simulink model "RLtrot"  (R2021b)
settings: Solver=ode15s  StartTime=0.0  StopTime=Tf  FixedStep=0.01  MaxStep=0.05  RelTol=0.5  AbsTol=0.5
model workspace (MATLAB code in the model file):
  | %---------------Critical values---------------%
  | angle_amp = pi/6; % Motor rotate amplitude, ref: pi/4
  | rotateCorrectionCoef = 1.158;
  | criticalFn = 2;
  | 
  | %------values for normalization---------------%
  | % values got by running manual gait
  | rotxNormGain = 1/0.1;
  | rotyNormGain = 1/0.05;
  | rotzNormGain = 1/0.1;
  | 
  | vxNormGain = 1/0.2;
  | vyNormGain = 1/0.2;
  | vzNormGain = 1/0.2;
  | 
  | FnNormGain = 1/15;
  | 
  | %--------values for check done---------------%
  | rotDone = 0.15;
  | legBendDone = pi/3; % actuator max bending angle
  | 
  | 
  | %---------------Robot parameters-------------%
  | % robot size
  | robot_width = 0.15;
  | robot_length = 0.22;
  | 
  | % floor parameters
  | floor_length = 2;
  | floor_width = 2;
  | 
  | % continuum actuator size
  | L_disk = 0.02944;% Disk side length (m)
  | R_w = L_disk/sqrt(3);
  | thickness_disk = 0.004; % Disk thickness (m)
  | thigh_length = 0.06;
  | R_core = 0.005; % Core radius (m)
  | length_core = 0.008; % Core length (m)
  | R_spool = 0.021; % 0.01944; % radius of the spool
  | spool_height = 0.022+0.015;
  | R_pulley = 1e-3;
  | spool_k = 0;
  | spool_d = 0;
  | hole_d = 4e-3;
  | 
  | % Material property
  | rho_PLA = 1.24e3;
  | rho = 1.19e3; % 1.19e3; % Density (kg/m^3)
  | % use rigid joints
  | Pz_stiff = 135000;
  | Pz_damping = 500;
  | S_stiff = 0.0239;
  | S_damping = 7.5e-5;
  | S_low_Bound = -20;
  | S_up_Bound = 20;
  | 
  | R_foot = 0.015; % foot radius (m)
  | 
  | % motor parameter
  | stall_T = 11.2; % 11.2 cm*kg, stall torque
  | t_60_deg = 0.2; % 0.09 s
  | V_nomrmal = 6; % corresponding normal voltage
  | Jr = 0.0001; %g*cm^2, robot inertia
  | 
  | % contact force
  | coef_static_friction = 0.315;
  | coef_dynamic_friction = 0.3;
  | crictic_velocity = 0.3; % m/s
  | contact_suf_stiff = 1000; % N/m
  | contact_suf_damp = 50; % N/(m/s)
  | contact_region_width = 2e-3; % m
  | spoolOpacity = 0;
  | tendonColor = [0.902 0.902 0.902];
  | tendonOpacity = 0.1;
  | 
  | % If use point masses
  | MMainFrame = 198; % g
  | MServoMotor = 50.55;
  | MMotorSupport = 12.1;
  | MSpool = 9.2;
  | 
  | % Robot total weight about 2 kg
  | MComposateLoad = 200;
  | 
  | MBuck = 40; % x2
  | MPCB_RPi = 141.3;
  | MLiBattery = 120; % x2
  | MPowerBank = 66.5;
  | isLoadVisible = 0.1;
  | 
  | 
  | MThigh = 26.7963;
  | MCore = 0.747699;
  | MDisk = 1.78642;
  | MFoot = 16.8232;
values from neighbouring files (symbols this model uses):
  Tf = 10    [longTest.m]    (also in singleTest.m)
  Ts = 0.05    [longTest.m]    (also in singleTest.m)
  x_norm_min = min(x,[],1)    [preprocessData.m]
  x_norm_range = max(x,[],1) - min(x,[],1)    [preprocessData.m]
  y_norm_min = min(y,[],1)    [preprocessData.m]
  y_norm_range = max(y,[],1) - min(y,[],1)    [preprocessData.m]
undefined symbols (not defined in the file or in its folder): alpha_b_gain, alpha_r_gain, EntropyList, EntropyWeightList, fnVariance, isCheckDone, isContactBoolean, isUseExtAct, rotVariance, speedVariance, startAgentTime, VRef, z_l_gain
libraries: simulink x8, rllib x1, deeplib x1
settings Model: Creator=Qinglei Ji  LastModifiedBy=4DLab5
settings SolverCC: AutoScaleAbsTol=off  MaxConsecutiveZCs=100  MaxConsecutiveMinStep=10  DaesscMode=Fast  AutoInsertRateTranBlk=on
settings ExplorerConfigSet: InternalSimMechanicsExplorerSettings="<ExplorerConfiguration><canonicalview>default</canonicalview><AnimationSetting><BasePlaybackSpeed>1.0</BasePlaybackSpeed><PlaybackSpeedFactor>1.0</PlaybackSpeedFactor></AnimationSetting><TilePanel><TileInfo><Tiles Columns=\"1\" Count=\"1\" Rows=\"1\"><Column Weight=\"1\"/><Row Weight=\"1\"/><Tile Height=\"1\" Width=\"1\" X=\"0\" Y=\"0\"/></Tiles></TileInfo><SceneInfo><SceneViewer><BGColor><R>0.60000002384185791</R><G>0.60000002384185791</G><B>0.60000002384185791</B></BGColor><Camera><DoPerspective>off</DoPerspective><Position><X>-18.8331461547739707</X><Y>25.880517186070815</Y><Z>26.8100820833696147</Z></Position><Center><X>0.29785977478998571</X><Y>-0.293010908258582892</Y><Z>-0.346783787749327221</Z></Center><Up><X>0.517886432622382209</X><Y>-0.40389178028612327</Y><Z>0.754098848111419029</Z></Up><ViewLimDist>1</ViewLimDist><YLim>0.421333194645766129</YLim><XLim>0.456755011894746488</XLim></Camera></SceneViewer></SceneInfo></TilePanel><MechEditorPanel><Cameras/><GfxPanelCameraMap/><VideoCreator><PlaybackSpeedRatio>1.0</PlaybackSpeedRatio><FrameRate>60</FrameRate><VideoFormat>MPEG-4</VideoFormat><FrameSize>auto</FrameSize></VideoCreator></MechEditorPanel></ExplorerConfiguration>"

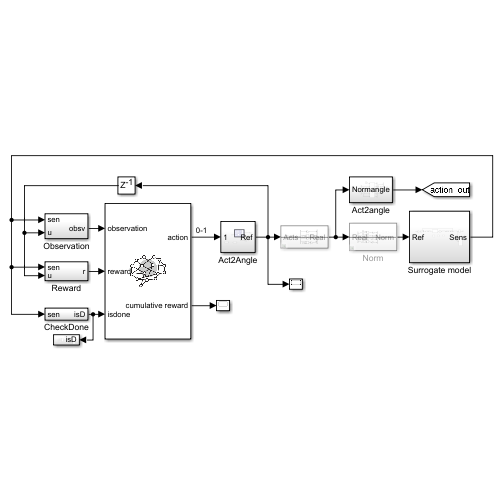
[thumbnail: Simulink's stored preview of the top-level diagram]
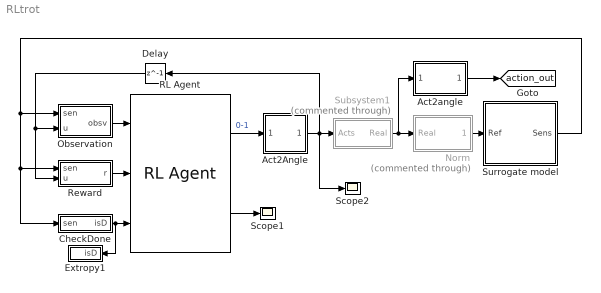
== system RLtrot ==
  Act2Angle : Subsystem
  Act2angle : Subsystem
  CheckDone : Subsystem
  Delay : Delay  DelayLength=1  InitialCondition=[0.5;0.5;0.5;0.5]
  Extropy1 : Subsystem
  Norm : Subsystem  Commented=through
  Observation : Subsystem
  RL Agent : rllib/RL Agent  Agent=agent  ExternalActionAsInput=off  ProvideCumRwd=on  TreatAsDirectFeedthrough=on
  Reward : Subsystem
  Scope1 : Scope
  Scope2 : Scope
  Subsystem1 : Subsystem  Commented=through
  Surrogate model : Subsystem
  tag scope: action_out=global
  wires:
  RL Agent/1 -> Act2Angle/1(In1)  "0-1"
  RL Agent/2 -> Scope1/1
  CheckDone/1(isD) -> Extropy1/1(isD), RL Agent/3
  Observation/1(obsv) -> RL Agent/1
  Reward/1(r) -> RL Agent/2
  Surrogate model/1(Sens) -> Observation/1(sen), Reward/1(sen), CheckDone/1(sen)
  Delay/1 -> Reward/2(u), Observation/2(u)
  Subsystem1/1(Real) -> Act2angle/1(Norm), Norm/1(Real)
  Act2Angle/1(Ref) -> Scope2/1, Delay/1, Subsystem1/1(Acts)
  Norm/1(Norm) -> Surrogate model/1(Ref)
  Act2angle/1(angle) -> [action_out]

== system RLtrot/Act2Angle ==
  note: Learn motor ref
  In1 : Inport
  DecideToUseExt : Subsystem
  Human expert : Subsystem
  Init : Subsystem
  Scope : Scope
  Subsystem2 : Subsystem  Commented=on
  action2angle : Subsystem  Commented=on
  useExt? : Switch  Criteria=u2 > Threshold
  Ref : Outport
  wires:
  In1/1 -> Init/1(In1)  "Acts"
  useExt?/1 -> Ref/1
  Human expert/1(Out1) -> useExt?/1
  DecideToUseExt/1(Out1) -> Scope/1, useExt?/2
  Init/1(Out1) -> useExt?/3

== system RLtrot/Act2angle ==
  Norm : Inport
  Demux : Demux
  MATLAB Function : MATLAB Function  TreatAsAtomicUnit=on
  MATLAB Function1 : MATLAB Function  TreatAsAtomicUnit=on
  Mux2 : Mux  Inputs=3
  Mux3 : Mux
  Mux4 : Mux  Inputs=3
  Subsystem : Subsystem
  alpha_r : Constant  Value=0
  alpha_r1 : Constant  Value=0
  angle : Outport
  wires:
  Mux2/1 -> Mux3/4, Mux3/2
  Mux4/1 -> Mux3/1, Mux3/3
  MATLAB Function1/1(alpha_A) -> Mux2/1
  MATLAB Function1/2(alpha_B) -> Mux2/2
  Mux3/1 -> angle/1  "ref"
  MATLAB Function/3(alpha_C) -> Mux4/3
  MATLAB Function/1(alpha_A) -> Mux4/1
  MATLAB Function/2(alpha_B) -> Mux4/2
  MATLAB Function1/3(alpha_C) -> Mux2/3
  alpha_r/1 -> MATLAB Function/1(alpha_r)
  alpha_r1/1 -> MATLAB Function1/1(alpha_r)
  Demux/1 -> MATLAB Function/2(alpha_b)  "b1"
  Demux/2 -> MATLAB Function/3(z_l)  "z1"
  Demux/3 -> MATLAB Function1/2(alpha_b)  "b2"
  Demux/4 -> MATLAB Function1/3(z_l)  "z2"
  Norm/1 -> Subsystem/1(Norm)
  Subsystem/1(Denorm) -> Demux/1

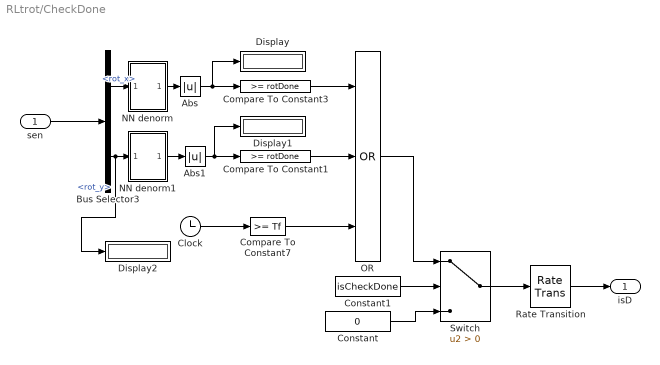
== system RLtrot/CheckDone ==
  sen : Inport
  Abs : Abs
  Abs1 : Abs
  Bus Selector3 : BusSelector  OutputSignals=rot_x,rot_y
  Clock : Clock
  Compare To Constant1 : simulink/Logic and Bit Operations/Compare To Constant  relop=>=  const=rotDone  OutDataTypeStr=boolean
  Compare To Constant3 : simulink/Logic and Bit Operations/Compare To Constant  relop=>=  const=rotDone  OutDataTypeStr=boolean
  Compare To Constant7 : simulink/Logic and Bit Operations/Compare To Constant  relop=>=  const=Tf  OutDataTypeStr=boolean
  Constant : Constant  Value=0
  Constant1 : Constant  Value=isCheckDone
  Display : Display
  Display1 : Display
  Display2 : Display
  NN denorm : Subsystem
  NN denorm1 : Subsystem
  OR : Logic  Operator=OR  Inputs=3  AllPortsSameDT=off  OutDataTypeStr=boolean
  Rate Transition : RateTransition
  Switch : Switch  Criteria=u2 > Threshold
  isD : Outport  VectorParamsAs1DForOutWhenUnconnected=off
  wires:
  sen/1 -> Bus Selector3/1
  Abs1/1 -> Display1/1, Compare To Constant1/1
  OR/1 -> Switch/1
  Compare To Constant7/1 -> OR/3
  Clock/1 -> Compare To Constant7/1
  Constant1/1 -> Switch/2
  Compare To Constant1/1 -> OR/2
  Abs/1 -> Display/1, Compare To Constant3/1
  Constant/1 -> Switch/3
  Switch/1 -> Rate Transition/1
  Compare To Constant3/1 -> OR/1
  Rate Transition/1 -> isD/1
  Bus Selector3/1 -> NN denorm/1(In1)  "<rot_x>"
  NN denorm/1(Out1) -> Abs/1
  Bus Selector3/2 -> Display2/1, NN denorm1/1(In1)  "<rot_y>"
  NN denorm1/1(Out1) -> Abs1/1

== system RLtrot/Extropy1 ==
  isD : Inport
  Clock : Clock
  Constant : Constant  Value=EntropyWeightList  SampleTime=Ts
  Constant2 : Constant  Value=EntropyList  SampleTime=Ts
  MATLAB Function : MATLAB Function  TreatAsAtomicUnit=on  SystemSampleTime=Ts
  MATLAB Function1 : MATLAB Function  TreatAsAtomicUnit=on
  wires:
  Constant2/1 -> MATLAB Function/2(EntropyList)  "entropy"
  Constant/1 -> MATLAB Function/1(EntropyWeightList)  "entroWeight"
  isD/1 -> MATLAB Function/3(isDone)
  [obsv_out] -> MATLAB Function1/2(obsv)
  [action_out] -> MATLAB Function1/3(act)
  Clock/1 -> MATLAB Function1/1(time)

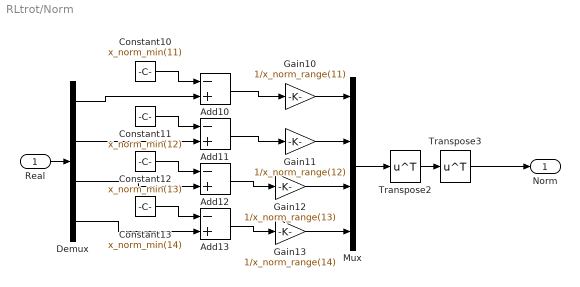
== system RLtrot/Norm ==
  Real : Inport
  Add{10..13} (4 alike) : Sum  Inputs=-+
  Constant10 : Constant  Value=x_norm_min(11)
  Constant11 : Constant  Value=x_norm_min(12)
  Constant12 : Constant  Value=x_norm_min(13)
  Constant13 : Constant  Value=x_norm_min(14)
  Demux : Demux
  Gain10 : Gain  Gain=1/x_norm_range(11)
  Gain11 : Gain  Gain=1/x_norm_range(12)
  Gain12 : Gain  Gain=1/x_norm_range(13)
  Gain13 : Gain  Gain=1/x_norm_range(14)
  Mux : Mux
  Transpose2 : Math  Operator=transpose  SaturateOnIntegerOverflow=on
  Transpose3 : Math  Operator=transpose  SaturateOnIntegerOverflow=on
  Norm : Outport
  wires:
  Constant10/1 -> Add10/1
  Constant11/1 -> Add11/1
  Demux/2 -> Add11/2
  Gain13/1 -> Mux/4
  Demux/4 -> Add13/2
  Add12/1 -> Gain12/1
  Demux/1 -> Add10/2
  Gain11/1 -> Mux/2
  Gain12/1 -> Mux/3
  Add11/1 -> Gain11/1
  Constant12/1 -> Add12/1
  Add10/1 -> Gain10/1
  Constant13/1 -> Add13/1
  Demux/3 -> Add12/2
  Add13/1 -> Gain13/1
  Gain10/1 -> Mux/1
  Real/1 -> Demux/1
  Transpose2/1 -> Transpose3/1
  Transpose3/1 -> Norm/1
  Mux/1 -> Transpose2/1

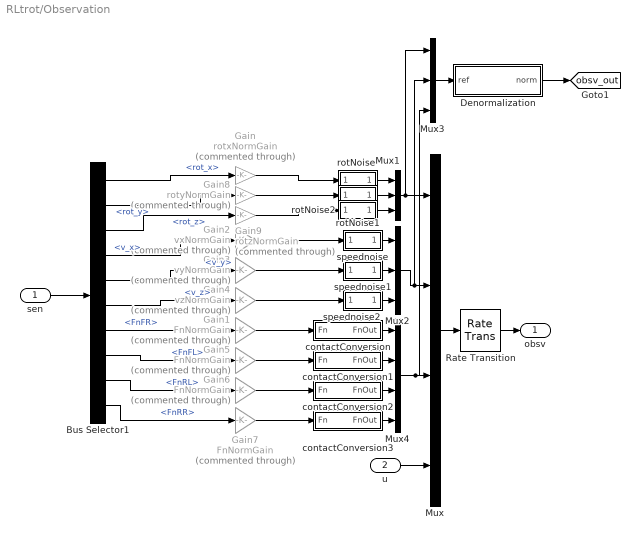
== system RLtrot/Observation ==
  sen : Inport
  u : Inport  Port=2
  Bus Selector1 : BusSelector  OutputSignals=rot_x,rot_y,rot_z,v_x,v_y,v_z,FnFR,FnFL,FnRL,FnRR
  Denormalization : Subsystem
  Gain : Gain  Commented=through  Gain=rotxNormGain
  Gain{1,5..7} (4 alike) : Gain  Commented=through  Gain=FnNormGain
  Gain2 : Gain  Commented=through  Gain=vxNormGain
  Gain3 : Gain  Commented=through  Gain=vyNormGain
  Gain4 : Gain  Commented=through  Gain=vzNormGain
  Gain8 : Gain  Commented=through  Gain=rotyNormGain
  Gain9 : Gain  Commented=through  Gain=rotzNormGain
  Mux : Mux
  Mux1 : Mux  Inputs=3
  Mux2 : Mux  Inputs=3
  Mux3 : Mux  Inputs=3
  Mux4 : Mux
  Rate Transition : RateTransition  OutPortSampleTime=Ts
  contactConversion : Subsystem
  contactConversion1 : Subsystem
  contactConversion2 : Subsystem
  contactConversion3 : Subsystem
  rotNoise : Subsystem
  rotNoise1 : Subsystem
  rotNoise2 : Subsystem
  speednoise : Subsystem
  speednoise1 : Subsystem
  speednoise2 : Subsystem
  obsv : Outport  VectorParamsAs1DForOutWhenUnconnected=off
  tag scope: obsv_out=global
  wires:
  Mux/1 -> Rate Transition/1
  sen/1 -> Bus Selector1/1
  Rate Transition/1 -> obsv/1
  u/1 -> Mux/4
  Mux1/1 -> Mux3/1, Mux/1
  Mux2/1 -> Mux3/2, Mux/2
  contactConversion/1(FnOut) -> Mux4/1
  contactConversion1/1(FnOut) -> Mux4/2
  contactConversion2/1(FnOut) -> Mux4/3
  contactConversion3/1(FnOut) -> Mux4/4
  Mux4/1 -> Mux3/3, Mux/3
  speednoise/1(Out1) -> Mux2/1
  speednoise1/1(Out1) -> Mux2/2
  speednoise2/1(Out1) -> Mux2/3
  Bus Selector1/1 -> Gain/1  "<rot_x>"
  rotNoise/1(Out1) -> Mux1/1
  rotNoise1/1(Out1) -> Mux1/2
  rotNoise2/1(Out1) -> Mux1/3
  Bus Selector1/2 -> Gain8/1  "<rot_y>"
  Bus Selector1/3 -> Gain9/1  "<rot_z>"
  Bus Selector1/4 -> Gain2/1  "<v_x>"
  Bus Selector1/5 -> Gain3/1  "<v_y>"
  Bus Selector1/6 -> Gain4/1  "<v_z>"
  Bus Selector1/7 -> Gain1/1  "<FnFR>"
  Bus Selector1/8 -> Gain5/1  "<FnFL>"
  Bus Selector1/9 -> Gain6/1  "<FnRL>"
  Bus Selector1/10 -> Gain7/1  "<FnRR>"
  Gain/1 -> rotNoise/1(<vx>)
  Gain8/1 -> rotNoise1/1(<vx>)
  Gain9/1 -> rotNoise2/1(<vx>)
  Gain2/1 -> speednoise/1(<vx>)
  Gain1/1 -> contactConversion/1(Fn)
  Gain6/1 -> contactConversion2/1(Fn)
  Gain5/1 -> contactConversion1/1(Fn)
  Gain3/1 -> speednoise1/1(<vx>)
  Gain4/1 -> speednoise2/1(<vx>)
  Gain7/1 -> contactConversion3/1(Fn)
  Denormalization/1(norm) -> [obsv_out]
  Mux3/1 -> Denormalization/1(ref)

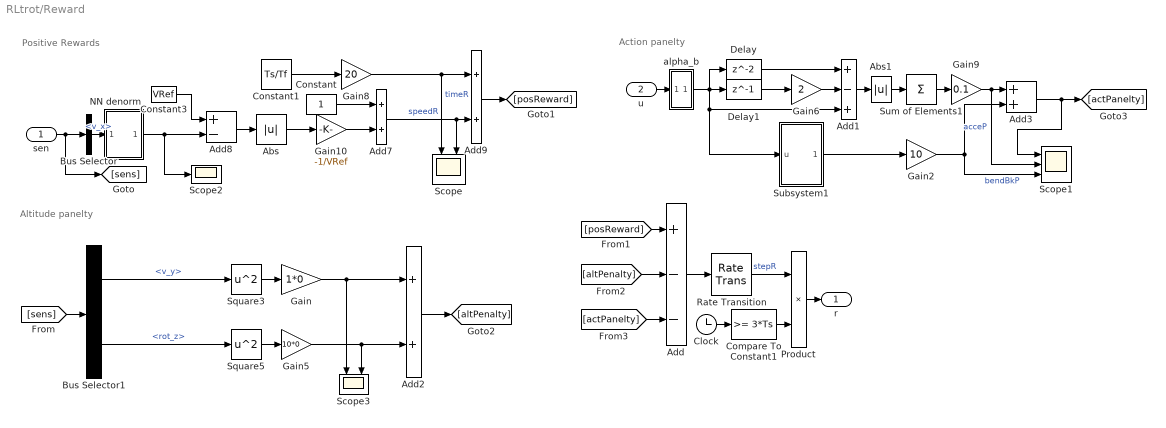
== system RLtrot/Reward ==
  note: Action panelty
  note: Altitude panelty
  note: Positive Rewards
  sen : Inport
  u : Inport  Port=2
  Abs : Abs
  Abs1 : Abs
  Add : Sum  Inputs=+--
  Add1 : Sum  Inputs=+-+
  Add{2..3,7,9} (4 alike) : Sum
  Add8 : Sum  Inputs=+-
  Bus Selector : BusSelector  OutputSignals=v_x
  Bus Selector1 : BusSelector  OutputSignals=v_y,rot_z
  Clock : Clock
  Compare To Constant1 : simulink/Logic and Bit Operations/Compare To Constant  relop=>=  const=3*Ts  OutDataTypeStr=boolean
  Constant : Constant
  Constant1 : Constant  Value=Ts/Tf
  Constant3 : Constant  Value=VRef
  Delay : Delay  InitialCondition=0.5
  Delay1 : Delay  DelayLength=1  InitialCondition=0.5
  Gain : Gain  Gain=1*0
  Gain10 : Gain  Gain=-1/VRef
  Gain2 : Gain  Gain=10
  Gain5 : Gain  Gain=10*0
  Gain6 : Gain  Gain=2
  Gain8 : Gain  Gain=20
  Gain9 : Gain  Gain=0.1
  NN denorm : Subsystem
  Product : Product
  Rate Transition : RateTransition  OutPortSampleTime=Ts
  Scope : Scope  NumInputPorts=2
  Scope1 : Scope  NumInputPorts=3
  Scope2 : Scope
  Scope3 : Scope  NumInputPorts=2
  Square3 : Math  Operator=square  SignedPower=on  SaturateOnIntegerOverflow=on
  Square5 : Math  Operator=square  SignedPower=on  SaturateOnIntegerOverflow=on
  Subsystem1 : Subsystem
  Sum of Elements1 : Sum  Inputs=+
  alpha_b : Subsystem
  r : Outport  VectorParamsAs1DForOutWhenUnconnected=off
  wires:
  sen/1 -> Bus Selector/1, [sens]
  Square3/1 -> Gain/1
  Square5/1 -> Gain5/1
  Bus Selector1/2 -> Square5/1  "<rot_z>"
  Gain/1 -> Scope3/1, Add2/1
  Add/1 -> Rate Transition/1
  Constant1/1 -> Gain8/1
  Delay/1 -> Add1/1
  Gain6/1 -> Add1/2
  Add1/1 -> Abs1/1
  Abs1/1 -> Sum of Elements1/1
  Delay1/1 -> Gain6/1
  Sum of Elements1/1 -> Gain9/1
  Clock/1 -> Compare To Constant1/1
  Compare To Constant1/1 -> Product/2
  Rate Transition/1 -> Product/1  "stepR"
  Product/1 -> r/1
  [sens] -> Bus Selector1/1
  Gain8/1 -> Add9/1, Scope/1  "timeR"
  Add9/1 -> [posReward]
  Bus Selector1/1 -> Square3/1  "<v_y>"
  Gain5/1 -> Add2/2, Scope3/2
  Add2/1 -> [altPenalty]
  [posReward] -> Add/1
  [altPenalty] -> Add/2
  [actPanelty] -> Add/3
  Add8/1 -> Abs/1
  Add7/1 -> Scope/2, Add9/2  "speedR"
  Gain10/1 -> Add7/2
  Abs/1 -> Gain10/1
  Constant/1 -> Add7/1
  Constant3/1 -> Add8/1
  Bus Selector/1 -> NN denorm/1(In1)  "<v_x>"
  NN denorm/1(Out1) -> Scope2/1, Add8/2
  Gain9/1 -> Scope1/2, Add3/1  "acceP"
  Add3/1 -> Scope1/1, [actPanelty]
  u/1 -> alpha_b/1(u)
  Subsystem1/1(Out1) -> Gain2/1
  Gain2/1 -> Add3/2, Scope1/3  "bendBkP"
  alpha_b/1(b) -> Add1/3, Subsystem1/1(u), Delay/1, Delay1/1

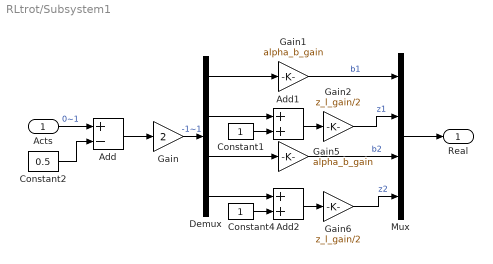
== system RLtrot/Subsystem1 ==
  Acts : Inport
  Add : Sum  Inputs=+-
  Add1 : Sum
  Add2 : Sum
  Constant1 : Constant
  Constant2 : Constant  Value=0.5
  Constant4 : Constant
  Demux : Demux
  Gain : Gain  Gain=2
  Gain1 : Gain  Gain=alpha_b_gain
  Gain2 : Gain  Gain=z_l_gain/2
  Gain5 : Gain  Gain=alpha_b_gain
  Gain6 : Gain  Gain=z_l_gain/2
  Mux : Mux
  Real : Outport
  wires:
  Demux/4 -> Add2/1
  Constant1/1 -> Add1/2
  Add1/1 -> Gain2/1
  Constant4/1 -> Add2/2
  Gain1/1 -> Mux/1  "b1"
  Acts/1 -> Add/1  "0~1"
  Constant2/1 -> Add/2
  Gain/1 -> Demux/1  "-1~1"
  Add2/1 -> Gain6/1
  Add/1 -> Gain/1
  Demux/1 -> Gain1/1
  Gain6/1 -> Mux/4  "z2"
  Mux/1 -> Real/1
  Gain2/1 -> Mux/2  "z1"
  Demux/2 -> Add1/1
  Demux/3 -> Gain5/1
  Gain5/1 -> Mux/3  "b2"

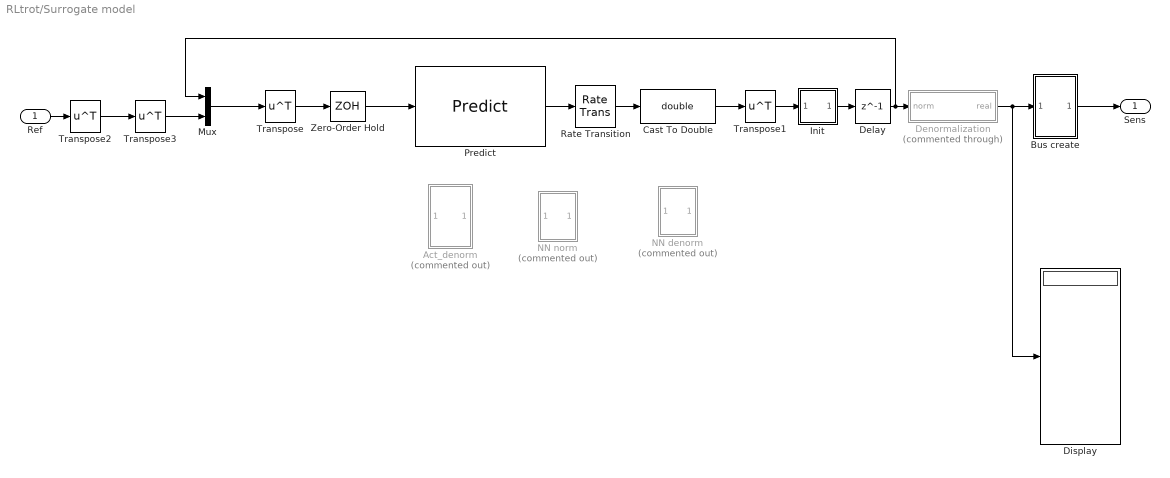
== system RLtrot/Surrogate model ==
  Ref : Inport
  Act_denorm : Subsystem  Commented=on
  Bus create : Subsystem
  Cast To Double : DataTypeConversion  OutDataTypeStr=double
  Delay : Delay  DelayLength=1  InitialCondition=x_norm_init'  SampleTime=Ts
  Denormalization : Subsystem  Commented=through
  Display : Display
  Init : Subsystem
  Mux : Mux  Inputs=2
  NN denorm : Subsystem  Commented=on
  NN norm : Subsystem  Commented=on
  Predict : deeplib/Predict  Network=Network from MAT-file  NetworkFunction=squeezenet  NetworkFilePath=C:\Users\4DLab5\OneDrive - KTH\KTH\Master Thesis\Github\MBRL23KTH\net_best.mat  MiniBatchSize=512  InputDataFormats={ 'observation', '[1x22]' }  Predictions=on  Activations={}  ForceInterpretedSim=off  EnableDLNetwork=on
      settings: SourceProductBaseCode=NN
  Rate Transition : RateTransition  OutPortSampleTime=Ts
  Transpose{,1..3} (4 alike) : Math  Operator=transpose  SaturateOnIntegerOverflow=on
  Zero-Order Hold : ZeroOrderHold  SampleTime=Ts
  Sens : Outport  OutDataTypeStr=double
  wires:
  Predict/1 -> Rate Transition/1
  Cast To Double/1 -> Transpose1/1
  Bus create/1(Outport) -> Sens/1
  Transpose/1 -> Zero-Order Hold/1
  Denormalization/1(real) -> Display/1, Bus create/1(In1)
  Mux/1 -> Transpose/1
  Init/1(Out1) -> Delay/1
  Transpose1/1 -> Init/1(In1)
  Delay/1 -> Mux/1, Denormalization/1(norm)
  Rate Transition/1 -> Cast To Double/1
  Zero-Order Hold/1 -> Predict/1
  Transpose2/1 -> Transpose3/1
  Transpose3/1 -> Mux/2
  Ref/1 -> Transpose2/1

== system RLtrot/Act2Angle/DecideToUseExt ==
  Clock : Clock
  Constant : Constant  Value=isUseExtAct
  Constant1 : Constant  Value=0
  Constant2 : Constant
  Constant3 : Constant  Value=0
  Switch : Switch  Criteria=u2 > Threshold  Threshold=startAgentTime
  Switch1 : Switch  Criteria=u2 > Threshold
  Out1 : Outport
  wires:
  Constant/1 -> Switch1/2
  Switch1/1 -> Out1/1
  Constant2/1 -> Switch/3
  Constant1/1 -> Switch/1
  Clock/1 -> Switch/2
  Constant3/1 -> Switch1/3
  Switch/1 -> Switch1/1

== system RLtrot/Act2Angle/Human expert ==
  Mux10 : Mux
  alpha_b : simulink/Sources/Repeating Sequence  rep_seq_t=[0 0.2 0.4 0.6 0.8]  rep_seq_y=[0.5 1 0.5 0 0.5]
  alpha_b1 : simulink/Sources/Repeating Sequence  rep_seq_t=[0 0.2 0.4 0.6 0.8]  rep_seq_y=[0.5 0 0.5 1 0.5]
  z_l : simulink/Sources/Repeating Sequence  rep_seq_t=[0 0.2 0.4 0.6 0.8]  rep_seq_y=[0 1 1 1 0]
  z_l1 : simulink/Sources/Repeating Sequence  rep_seq_t=[0 0.2 0.4 0.6 0.8]  rep_seq_y=[1 1 0 1 1]
  Out1 : Outport
  wires:
  Mux10/1 -> Out1/1
  alpha_b/1 -> Mux10/1  "alpha_b_Ref"
  z_l1/1 -> Mux10/4  "z_l_Ref"
  z_l/1 -> Mux10/2  "z_l_Ref"
  alpha_b1/1 -> Mux10/3  "alpha_b_Ref"

== system RLtrot/Act2Angle/Init ==
  In1 : Inport
  Clock : Clock
  Constant{6..9} (4 alike) : Constant  Value=0.5
  Initial : Switch  Threshold=Ts
  Mux : Mux
  Out1 : Outport
  wires:
  Mux/1 -> Initial/3
  In1/1 -> Initial/1
  Initial/1 -> Out1/1  "prosedAct"
  Clock/1 -> Initial/2
  Constant9/1 -> Mux/4
  Constant6/1 -> Mux/1
  Constant8/1 -> Mux/3
  Constant7/1 -> Mux/2

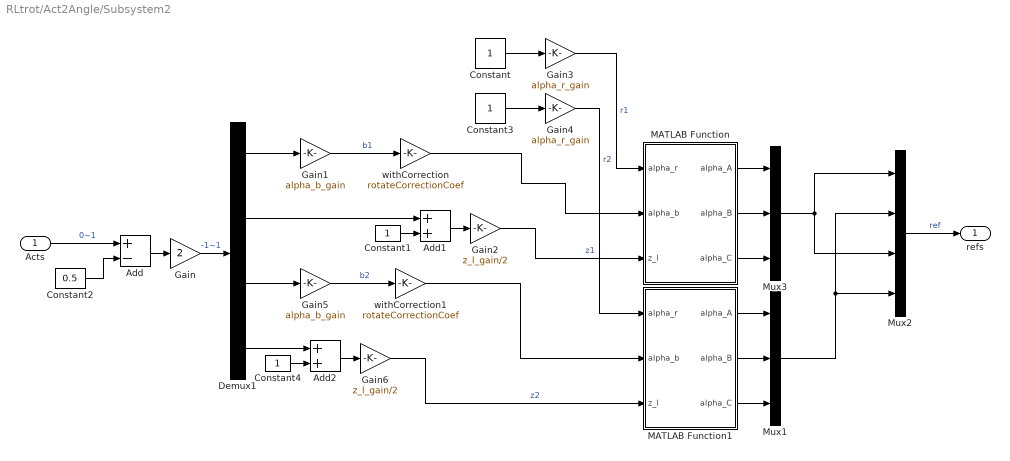
== system RLtrot/Act2Angle/Subsystem2 ==
  Acts : Inport
  Add : Sum  Inputs=+-
  Add1 : Sum
  Add2 : Sum
  Constant{,1,3..4} (4 alike) : Constant
  Constant2 : Constant  Value=0.5
  Demux1 : Demux
  Gain : Gain  Gain=2
  Gain1 : Gain  Gain=alpha_b_gain
  Gain2 : Gain  Gain=z_l_gain/2
  Gain3 : Gain  Gain=alpha_r_gain
  Gain4 : Gain  Gain=alpha_r_gain
  Gain5 : Gain  Gain=alpha_b_gain
  Gain6 : Gain  Gain=z_l_gain/2
  MATLAB Function : MATLAB Function  TreatAsAtomicUnit=on
  MATLAB Function1 : MATLAB Function  TreatAsAtomicUnit=on
  Mux1 : Mux  Inputs=3
  Mux2 : Mux
  Mux3 : Mux  Inputs=3
  withCorrection : Gain  Gain=rotateCorrectionCoef
  withCorrection1 : Gain  Gain=rotateCorrectionCoef
  refs : Outport
  wires:
  Gain6/1 -> MATLAB Function1/3(z_l)  "z2"
  Mux2/1 -> refs/1  "ref"
  Gain2/1 -> MATLAB Function/3(z_l)  "z1"
  Gain4/1 -> MATLAB Function1/1(alpha_r)  "r2"
  MATLAB Function1/1(alpha_A) -> Mux1/1
  Gain3/1 -> MATLAB Function/1(alpha_r)  "r1"
  Gain1/1 -> withCorrection/1  "b1"
  MATLAB Function/3(alpha_C) -> Mux3/3
  MATLAB Function1/3(alpha_C) -> Mux1/3
  MATLAB Function/1(alpha_A) -> Mux3/1
  MATLAB Function/2(alpha_B) -> Mux3/2
  MATLAB Function1/2(alpha_B) -> Mux1/2
  Mux3/1 -> Mux2/1, Mux2/3
  Mux1/1 -> Mux2/4, Mux2/2
  Demux1/1 -> Gain1/1
  Constant/1 -> Gain3/1
  Constant3/1 -> Gain4/1
  Constant1/1 -> Add1/2
  Add1/1 -> Gain2/1
  Gain5/1 -> withCorrection1/1  "b2"
  Demux1/4 -> Add2/1
  Add2/1 -> Gain6/1
  Constant4/1 -> Add2/2
  withCorrection/1 -> MATLAB Function/2(alpha_b)
  withCorrection1/1 -> MATLAB Function1/2(alpha_b)
  Constant2/1 -> Add/2
  Acts/1 -> Add/1  "0~1"
  Add/1 -> Gain/1
  Gain/1 -> Demux1/1  "-1~1"
  Demux1/2 -> Add1/1
  Demux1/3 -> Gain5/1

== system RLtrot/Act2Angle/action2angle ==
  In1 : Inport
  Add : Sum  Inputs=+-
  Constant2 : Constant  Value=0.5
  withCorrection : Gain  Gain=angle_amp/0.5*rotateCorrectionCoef
  currAct_vec : Outport
  wires:
  In1/1 -> Add/1
  Constant2/1 -> Add/2
  Add/1 -> withCorrection/1
  withCorrection/1 -> currAct_vec/1

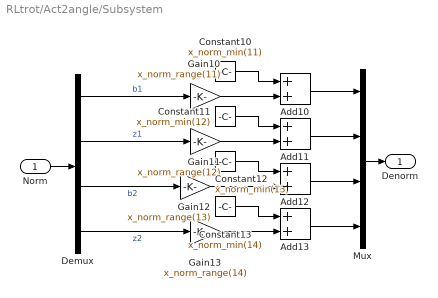
== system RLtrot/Act2angle/Subsystem ==
  Norm : Inport
  Add{10..13} (4 alike) : Sum
  Constant10 : Constant  Value=x_norm_min(11)
  Constant11 : Constant  Value=x_norm_min(12)
  Constant12 : Constant  Value=x_norm_min(13)
  Constant13 : Constant  Value=x_norm_min(14)
  Demux : Demux
  Gain10 : Gain  Gain=x_norm_range(11)
  Gain11 : Gain  Gain=x_norm_range(12)
  Gain12 : Gain  Gain=x_norm_range(13)
  Gain13 : Gain  Gain=x_norm_range(14)
  Mux : Mux
  Denorm : Outport
  wires:
  Constant12/1 -> Add12/1
  Add13/1 -> Mux/4
  Gain10/1 -> Add10/2
  Gain11/1 -> Add11/2
  Demux/1 -> Gain10/1  "b1"
  Add11/1 -> Mux/2
  Demux/3 -> Gain12/1  "b2"
  Gain13/1 -> Add13/2
  Gain12/1 -> Add12/2
  Constant13/1 -> Add13/1
  Mux/1 -> Denorm/1
  Demux/4 -> Gain13/1  "z2"
  Add10/1 -> Mux/1
  Add12/1 -> Mux/3
  Constant11/1 -> Add11/1
  Demux/2 -> Gain11/1  "z1"
  Constant10/1 -> Add10/1
  Norm/1 -> Demux/1

== system RLtrot/CheckDone/NN denorm ==
  In1 : Inport
  0~1to-1~1s : Subsystem  Commented=through
  Add : Sum
  Constant : Constant  Value=y_norm_min(1)  SampleTime=Ts
  Gain : Gain  Gain=y_norm_range(1)
  Out1 : Outport
  wires:
  Constant/1 -> Add/2
  Add/1 -> Out1/1
  Gain/1 -> Add/1
  In1/1 -> 0~1to-1~1s/1(In1)
  0~1to-1~1s/1(Out1) -> Gain/1

== system RLtrot/CheckDone/NN denorm1 ==
  In1 : Inport
  0~1to-1~1s : Subsystem  Commented=through
  Add : Sum
  Constant : Constant  Value=y_norm_min(2)  SampleTime=Ts
  Gain : Gain  Gain=y_norm_range(2)
  Out1 : Outport
  wires:
  Constant/1 -> Add/2
  Add/1 -> Out1/1
  Gain/1 -> Add/1
  In1/1 -> 0~1to-1~1s/1(In1)
  0~1to-1~1s/1(Out1) -> Gain/1

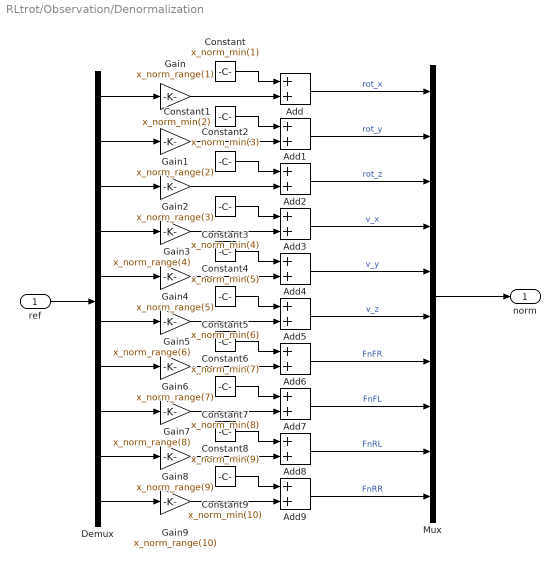
== system RLtrot/Observation/Denormalization ==
  ref : Inport
  Add{,1..9} (10 alike) : Sum
  Constant : Constant  Value=x_norm_min(1)
  Constant1 : Constant  Value=x_norm_min(2)
  Constant2 : Constant  Value=x_norm_min(3)
  Constant3 : Constant  Value=x_norm_min(4)
  Constant4 : Constant  Value=x_norm_min(5)
  Constant5 : Constant  Value=x_norm_min(6)
  Constant6 : Constant  Value=x_norm_min(7)
  Constant7 : Constant  Value=x_norm_min(8)
  Constant8 : Constant  Value=x_norm_min(9)
  Constant9 : Constant  Value=x_norm_min(10)
  Demux : Demux  Outputs=10
  Gain : Gain  Gain=x_norm_range(1)
  Gain1 : Gain  Gain=x_norm_range(2)
  Gain2 : Gain  Gain=x_norm_range(3)
  Gain3 : Gain  Gain=x_norm_range(4)
  Gain4 : Gain  Gain=x_norm_range(5)
  Gain5 : Gain  Gain=x_norm_range(6)
  Gain6 : Gain  Gain=x_norm_range(7)
  Gain7 : Gain  Gain=x_norm_range(8)
  Gain8 : Gain  Gain=x_norm_range(9)
  Gain9 : Gain  Gain=x_norm_range(10)
  Mux : Mux  Inputs=10
  norm : Outport
  wires:
  Mux/1 -> norm/1
  ref/1 -> Demux/1
  Constant/1 -> Add/1
  Constant1/1 -> Add1/1
  Constant2/1 -> Add2/1
  Constant3/1 -> Add3/1
  Constant4/1 -> Add4/1
  Constant5/1 -> Add5/1
  Constant6/1 -> Add6/1
  Constant7/1 -> Add7/1
  Constant8/1 -> Add8/1
  Constant9/1 -> Add9/1
  Demux/1 -> Gain/1
  Demux/2 -> Gain1/1
  Demux/3 -> Gain2/1
  Demux/4 -> Gain3/1
  Demux/5 -> Gain4/1
  Demux/6 -> Gain5/1
  Demux/7 -> Gain6/1
  Demux/8 -> Gain7/1
  Demux/9 -> Gain8/1
  Demux/10 -> Gain9/1
  Gain9/1 -> Add9/2
  Gain/1 -> Add/2
  Gain1/1 -> Add1/2
  Gain2/1 -> Add2/2
  Gain3/1 -> Add3/2
  Gain4/1 -> Add4/2
  Gain5/1 -> Add5/2
  Gain6/1 -> Add6/2
  Gain7/1 -> Add7/2
  Gain8/1 -> Add8/2
  Add/1 -> Mux/1  "rot_x"
  Add1/1 -> Mux/2  "rot_y"
  Add2/1 -> Mux/3  "rot_z"
  Add3/1 -> Mux/4  "v_x"
  Add9/1 -> Mux/10  "FnRR"
  Add8/1 -> Mux/9  "FnRL"
  Add7/1 -> Mux/8  "FnFL"
  Add6/1 -> Mux/7  "FnFR"
  Add5/1 -> Mux/6  "v_z"
  Add4/1 -> Mux/5  "v_y"

== system RLtrot/Observation/contactConversion ==
  Fn : Inport
  Constant : Constant  Value=isContactBoolean
  Constant1 : Constant
  Constant2 : Constant  Value=0
  Switch : Switch  Criteria=u2 > Threshold  Threshold=criticalFn*FnNormGain
  Switch1 : Switch  Criteria=u2 > Threshold
  fnNoise : Subsystem
  FnOut : Outport
  wires:
  Fn/1 -> fnNoise/1(<vx>)
  Constant/1 -> Switch1/2
  Constant2/1 -> Switch/3
  Constant1/1 -> Switch/1
  Switch/1 -> Switch1/1
  Switch1/1 -> FnOut/1
  fnNoise/1(Out1) -> Switch/2, Switch1/3

== system RLtrot/Observation/contactConversion1 ==
  Fn : Inport
  Constant : Constant  Value=isContactBoolean
  Constant1 : Constant
  Constant2 : Constant  Value=0
  Switch : Switch  Criteria=u2 > Threshold  Threshold=criticalFn*FnNormGain
  Switch1 : Switch  Criteria=u2 > Threshold
  fnNoise : Subsystem
  FnOut : Outport
  wires:
  Fn/1 -> fnNoise/1(<vx>)
  Constant/1 -> Switch1/2
  Constant2/1 -> Switch/3
  Constant1/1 -> Switch/1
  Switch/1 -> Switch1/1
  Switch1/1 -> FnOut/1
  fnNoise/1(Out1) -> Switch/2, Switch1/3

== system RLtrot/Observation/contactConversion2 ==
  Fn : Inport
  Constant : Constant  Value=isContactBoolean
  Constant1 : Constant
  Constant2 : Constant  Value=0
  Switch : Switch  Criteria=u2 > Threshold  Threshold=criticalFn*FnNormGain
  Switch1 : Switch  Criteria=u2 > Threshold
  fnNoise : Subsystem
  FnOut : Outport
  wires:
  Fn/1 -> fnNoise/1(<vx>)
  Constant/1 -> Switch1/2
  Constant2/1 -> Switch/3
  Constant1/1 -> Switch/1
  Switch/1 -> Switch1/1
  Switch1/1 -> FnOut/1
  fnNoise/1(Out1) -> Switch/2, Switch1/3

== system RLtrot/Observation/contactConversion3 ==
  Fn : Inport
  Constant : Constant  Value=isContactBoolean
  Constant1 : Constant
  Constant2 : Constant  Value=0
  Switch : Switch  Criteria=u2 > Threshold  Threshold=criticalFn*FnNormGain
  Switch1 : Switch  Criteria=u2 > Threshold
  fnNoise : Subsystem
  FnOut : Outport
  wires:
  Fn/1 -> fnNoise/1(<vx>)
  Constant/1 -> Switch1/2
  Constant2/1 -> Switch/3
  Constant1/1 -> Switch/1
  Switch/1 -> Switch1/1
  Switch1/1 -> FnOut/1
  fnNoise/1(Out1) -> Switch/2, Switch1/3

== system RLtrot/Observation/rotNoise ==
  <vx> : Inport
  Add : Sum
  Random Number : RandomNumber  Variance=rotVariance  SampleTime=Ts
  Out1 : Outport
  wires:
  Random Number/1 -> Add/1
  <vx>/1 -> Add/2
  Add/1 -> Out1/1

== system RLtrot/Observation/rotNoise1 ==
  <vx> : Inport
  Add : Sum
  Random Number : RandomNumber  Variance=rotVariance  Seed=1  SampleTime=Ts
  Out1 : Outport
  wires:
  Random Number/1 -> Add/1
  <vx>/1 -> Add/2
  Add/1 -> Out1/1

== system RLtrot/Observation/rotNoise2 ==
  <vx> : Inport
  Add : Sum
  Random Number : RandomNumber  Variance=rotVariance  Seed=12  SampleTime=Ts
  Out1 : Outport
  wires:
  Random Number/1 -> Add/1
  <vx>/1 -> Add/2
  Add/1 -> Out1/1

== system RLtrot/Observation/speednoise ==
  <vx> : Inport
  Add : Sum
  Random Number : RandomNumber  Variance=speedVariance  Seed=3  SampleTime=Ts
  Out1 : Outport
  wires:
  Random Number/1 -> Add/1
  <vx>/1 -> Add/2
  Add/1 -> Out1/1

== system RLtrot/Observation/speednoise1 ==
  <vx> : Inport
  Add : Sum
  Random Number : RandomNumber  Variance=speedVariance  Seed=4  SampleTime=Ts
  Out1 : Outport
  wires:
  Random Number/1 -> Add/1
  <vx>/1 -> Add/2
  Add/1 -> Out1/1

== system RLtrot/Observation/speednoise2 ==
  <vx> : Inport
  Add : Sum
  Random Number : RandomNumber  Variance=speedVariance  Seed=5  SampleTime=Ts
  Out1 : Outport
  wires:
  Random Number/1 -> Add/1
  <vx>/1 -> Add/2
  Add/1 -> Out1/1

== system RLtrot/Reward/NN denorm ==
  In1 : Inport
  Add : Sum
  Constant : Constant  Value=y_norm_min(4)  SampleTime=Ts
  Gain : Gain  Gain=y_norm_range(4)
  Out1 : Outport
  wires:
  Constant/1 -> Add/2
  Add/1 -> Out1/1
  Gain/1 -> Add/1
  In1/1 -> Gain/1

== system RLtrot/Reward/Subsystem1 ==
  u : Inport
  Abs1 : Abs
  Add : Sum
  Add1 : Sum  Inputs=+-
  Add2 : Sum  Inputs=+-
  Constant : Constant  Value=2*0.35
  Constant1 : Constant  Value=4*0.36
  Constant2 : Constant  Value=0
  Demux : Demux  Outputs=2
  Math Function : Math  Operator=square  SaturateOnIntegerOverflow=on
  Max : MinMax  Function=max  Inputs=2
  Out1 : Outport
  wires:
  Math Function/1 -> Out1/1
  u/1 -> Demux/1
  Demux/1 -> Add/1  "b1"
  Demux/2 -> Add/2  "b2"
  Add/1 -> Add1/1
  Constant/1 -> Add1/2
  Add1/1 -> Abs1/1
  Abs1/1 -> Add2/1
  Constant1/1 -> Add2/2
  Add2/1 -> Max/1
  Constant2/1 -> Max/2
  Max/1 -> Math Function/1

== system RLtrot/Reward/alpha_b ==
  u : Inport
  Demux : Demux
  Mux : Mux  Inputs=2
  Terminator : Terminator
  Terminator1 : Terminator
  b : Outport
  wires:
  Demux/3 -> Mux/2  "b2"
  Demux/1 -> Mux/1  "b1"
  Demux/2 -> Terminator/1  "z1"
  Mux/1 -> b/1
  u/1 -> Demux/1
  Demux/4 -> Terminator1/1  "z2"

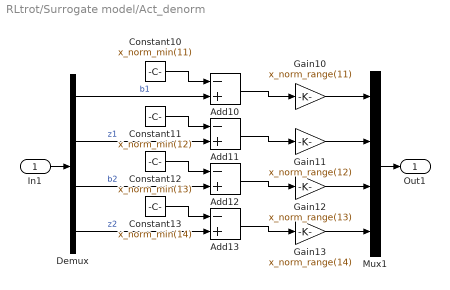
== system RLtrot/Surrogate model/Act_denorm ==
  In1 : Inport
  Add{10..13} (4 alike) : Sum  Inputs=-+
  Constant10 : Constant  Value=x_norm_min(11)
  Constant11 : Constant  Value=x_norm_min(12)
  Constant12 : Constant  Value=x_norm_min(13)
  Constant13 : Constant  Value=x_norm_min(14)
  Demux : Demux
  Gain10 : Gain  Gain=x_norm_range(11)
  Gain11 : Gain  Gain=x_norm_range(12)
  Gain12 : Gain  Gain=x_norm_range(13)
  Gain13 : Gain  Gain=x_norm_range(14)
  Mux1 : Mux
  Out1 : Outport
  wires:
  Gain11/1 -> Mux1/2
  Gain13/1 -> Mux1/4
  Gain10/1 -> Mux1/1
  Gain12/1 -> Mux1/3
  Demux/3 -> Add12/2  "b2"
  Mux1/1 -> Out1/1
  Demux/2 -> Add11/2  "z1"
  In1/1 -> Demux/1
  Demux/4 -> Add13/2  "z2"
  Demux/1 -> Add10/2  "b1"
  Add12/1 -> Gain12/1
  Constant13/1 -> Add13/1
  Add13/1 -> Gain13/1
  Add10/1 -> Gain10/1
  Constant11/1 -> Add11/1
  Constant12/1 -> Add12/1
  Add11/1 -> Gain11/1
  Constant10/1 -> Add10/1

== system RLtrot/Surrogate model/Bus create ==
  In1 : Inport
  Bus Creator : BusCreator  Inputs=10
  Demux : Demux  Outputs=10
  Outport : Outport
  wires:
  In1/1 -> Demux/1
  Demux/1 -> Bus Creator/1  "rot_x"
  Demux/2 -> Bus Creator/2  "rot_y"
  Demux/3 -> Bus Creator/3  "rot_z"
  Bus Creator/1 -> Outport/1
  Demux/4 -> Bus Creator/4  "v_x"
  Demux/5 -> Bus Creator/5  "v_y"
  Demux/6 -> Bus Creator/6  "v_z"
  Demux/7 -> Bus Creator/7  "FnFR"
  Demux/8 -> Bus Creator/8  "FnFL"
  Demux/9 -> Bus Creator/9  "FnRL"
  Demux/10 -> Bus Creator/10  "FnRR"

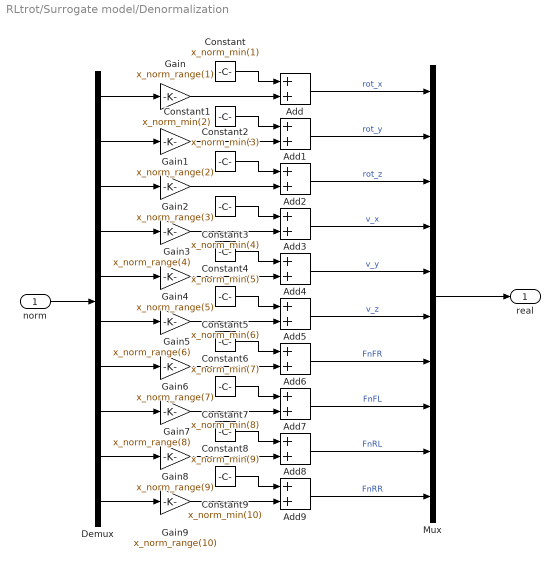
== system RLtrot/Surrogate model/Denormalization ==
  norm : Inport
  Add{,1..9} (10 alike) : Sum
  Constant : Constant  Value=x_norm_min(1)
  Constant1 : Constant  Value=x_norm_min(2)
  Constant2 : Constant  Value=x_norm_min(3)
  Constant3 : Constant  Value=x_norm_min(4)
  Constant4 : Constant  Value=x_norm_min(5)
  Constant5 : Constant  Value=x_norm_min(6)
  Constant6 : Constant  Value=x_norm_min(7)
  Constant7 : Constant  Value=x_norm_min(8)
  Constant8 : Constant  Value=x_norm_min(9)
  Constant9 : Constant  Value=x_norm_min(10)
  Demux : Demux  Outputs=10
  Gain : Gain  Gain=x_norm_range(1)
  Gain1 : Gain  Gain=x_norm_range(2)
  Gain2 : Gain  Gain=x_norm_range(3)
  Gain3 : Gain  Gain=x_norm_range(4)
  Gain4 : Gain  Gain=x_norm_range(5)
  Gain5 : Gain  Gain=x_norm_range(6)
  Gain6 : Gain  Gain=x_norm_range(7)
  Gain7 : Gain  Gain=x_norm_range(8)
  Gain8 : Gain  Gain=x_norm_range(9)
  Gain9 : Gain  Gain=x_norm_range(10)
  Mux : Mux  Inputs=10
  real : Outport
  wires:
  Mux/1 -> real/1
  norm/1 -> Demux/1
  Constant/1 -> Add/1
  Constant1/1 -> Add1/1
  Constant2/1 -> Add2/1
  Constant3/1 -> Add3/1
  Constant4/1 -> Add4/1
  Constant5/1 -> Add5/1
  Constant6/1 -> Add6/1
  Constant7/1 -> Add7/1
  Constant8/1 -> Add8/1
  Constant9/1 -> Add9/1
  Demux/1 -> Gain/1
  Demux/2 -> Gain1/1
  Demux/3 -> Gain2/1
  Demux/4 -> Gain3/1
  Demux/5 -> Gain4/1
  Demux/6 -> Gain5/1
  Demux/7 -> Gain6/1
  Demux/8 -> Gain7/1
  Demux/9 -> Gain8/1
  Demux/10 -> Gain9/1
  Gain9/1 -> Add9/2
  Gain/1 -> Add/2
  Gain1/1 -> Add1/2
  Gain2/1 -> Add2/2
  Gain3/1 -> Add3/2
  Gain4/1 -> Add4/2
  Gain5/1 -> Add5/2
  Gain6/1 -> Add6/2
  Gain7/1 -> Add7/2
  Gain8/1 -> Add8/2
  Add/1 -> Mux/1  "rot_x"
  Add1/1 -> Mux/2  "rot_y"
  Add2/1 -> Mux/3  "rot_z"
  Add3/1 -> Mux/4  "v_x"
  Add9/1 -> Mux/10  "FnRR"
  Add8/1 -> Mux/9  "FnRL"
  Add7/1 -> Mux/8  "FnFL"
  Add6/1 -> Mux/7  "FnFR"
  Add5/1 -> Mux/6  "v_z"
  Add4/1 -> Mux/5  "v_y"

== system RLtrot/Surrogate model/Init ==
  In1 : Inport
  0 : Subsystem
  Clock : Clock
  Display : Display
  Initial : Switch  Threshold=Ts
  real : Subsystem
  Out1 : Outport
  wires:
  In1/1 -> Initial/1
  Initial/1 -> Out1/1  "prosedAct"
  Clock/1 -> Initial/2
  real/1(Out1) -> Display/1, Initial/3

== system RLtrot/Surrogate model/NN denorm ==
  In1 : Inport
  Add : Sum
  Constant : Constant  Value=y_norm_min  SampleTime=Ts
  Gain : Gain  Gain=y_norm_range'
  Out1 : Outport
  wires:
  Constant/1 -> Add/2
  Add/1 -> Out1/1
  Gain/1 -> Add/1
  In1/1 -> Gain/1

== system RLtrot/Surrogate model/NN norm ==
  In1 : Inport
  Add : Sum  Inputs=+-
  Constant : Constant  Value=x_norm_min  SampleTime=Ts
  Gain : Gain  Gain=1./x_norm_range
  Transpose : Math  Operator=transpose  SaturateOnIntegerOverflow=on
  Transpose1 : Math  Operator=transpose  SaturateOnIntegerOverflow=on
  Out1 : Outport
  wires:
  Constant/1 -> Add/2
  Add/1 -> Gain/1
  Gain/1 -> Out1/1
  In1/1 -> Transpose/1
  Transpose/1 -> Transpose1/1
  Transpose1/1 -> Add/1

== system RLtrot/CheckDone/NN denorm/0~1to-1~1s ==
  In1 : Inport
  Add : Sum  Inputs=+-
  Constant : Constant  Value=0.5  SampleTime=Ts
  Gain : Gain  Gain=2
  Out1 : Outport
  wires:
  Gain/1 -> Out1/1
  Constant/1 -> Add/2
  Add/1 -> Gain/1
  In1/1 -> Add/1

== system RLtrot/CheckDone/NN denorm1/0~1to-1~1s ==
  In1 : Inport
  Add : Sum  Inputs=+-
  Constant : Constant  Value=0.5  SampleTime=Ts
  Gain : Gain  Gain=2
  Out1 : Outport
  wires:
  Gain/1 -> Out1/1
  Constant/1 -> Add/2
  Add/1 -> Gain/1
  In1/1 -> Add/1

== system RLtrot/Observation/contactConversion/fnNoise ==
  <vx> : Inport
  Add : Sum
  Random Number : RandomNumber  Variance=fnVariance  Seed=7  SampleTime=Ts
  Out1 : Outport
  wires:
  Random Number/1 -> Add/1
  <vx>/1 -> Add/2
  Add/1 -> Out1/1

== system RLtrot/Observation/contactConversion1/fnNoise ==
  <vx> : Inport
  Add : Sum
  Random Number : RandomNumber  Variance=fnVariance  Seed=8  SampleTime=Ts
  Out1 : Outport
  wires:
  Random Number/1 -> Add/1
  <vx>/1 -> Add/2
  Add/1 -> Out1/1

== system RLtrot/Observation/contactConversion2/fnNoise ==
  <vx> : Inport
  Add : Sum
  Random Number : RandomNumber  Variance=fnVariance  Seed=9  SampleTime=Ts
  Out1 : Outport
  wires:
  Random Number/1 -> Add/1
  <vx>/1 -> Add/2
  Add/1 -> Out1/1

== system RLtrot/Observation/contactConversion3/fnNoise ==
  <vx> : Inport
  Add : Sum
  Random Number : RandomNumber  Variance=fnVariance  Seed=10  SampleTime=Ts
  Out1 : Outport
  wires:
  Random Number/1 -> Add/1
  <vx>/1 -> Add/2
  Add/1 -> Out1/1

== system RLtrot/Surrogate model/Init/0 ==
  Constant{,1..5} (6 alike) : Constant  Commented=on  Value=0
  Constant{6..9} (4 alike) : Constant  Commented=on  Value=0.5
  Mux1 : Mux  Inputs=10
  Out1 : Outport
  wires:
  Constant8/1 -> Mux1/9
  Constant4/1 -> Mux1/5
  Constant3/1 -> Mux1/3
  Constant9/1 -> Mux1/10
  Constant/1 -> Mux1/1
  Constant1/1 -> Mux1/4
  Constant2/1 -> Mux1/2
  Constant6/1 -> Mux1/7
  Mux1/1 -> Out1/1
  Constant7/1 -> Mux1/8
  Constant5/1 -> Mux1/6

== system RLtrot/Surrogate model/Init/real ==
  Constant10 : Constant  Value=0.498915184272592
  Constant11 : Constant  Value=0.519835461568877
  Constant12 : Constant  Value=0.613462367245480
  Constant13 : Constant  Value=0.497839423077561
  Constant14 : Constant  Value=0.500037600573568
  Constant15 : Constant  Value=0.382025999336030
  Constant16 : Constant  Value=0.0297369618616698
  Constant17 : Constant  Value=0.0297303339285974
  Constant18 : Constant  Value=0.0263066122402123
  Constant19 : Constant  Value=0.0239024731524039
  Mux : Mux  Inputs=10
  Out1 : Outport
  wires:
  Constant16/1 -> Mux/7
  Constant12/1 -> Mux/2
  Constant19/1 -> Mux/10
  Constant14/1 -> Mux/5
  Constant13/1 -> Mux/3
  Constant11/1 -> Mux/4
  Constant15/1 -> Mux/6
  Constant10/1 -> Mux/1
  Constant17/1 -> Mux/8
  Constant18/1 -> Mux/9
  Mux/1 -> Out1/1

== matlab function RLtrot/Act2angle/MATLAB Function ==
  data: alpha_r input; alpha_A output; alpha_b input; z_l input; alpha_B output; alpha_C output
function [alpha_A, alpha_B, alpha_C]= fcn(alpha_r, alpha_b, z_l)

L_disk = 0.02944;% Disk side length (m)
R_spool = 0.021;
R_w = L_disk/sqrt(3);

alpha_A = (-R_w*alpha_b*cos(-alpha_r)+z_l)/R_spool;
alpha_B = (-R_w*alpha_b*cos(-alpha_r+2*pi/3)+z_l)/R_spool;
alpha_C = (-R_w*alpha_b*cos(-alpha_r+4*pi/3)+z_l)/R_spool;

== matlab function RLtrot/Act2Angle/Subsystem2/MATLAB Function ==
  data: alpha_r input; alpha_A output; alpha_b input; z_l input; alpha_B output; alpha_C output
function [alpha_A, alpha_B, alpha_C]= fcn(alpha_r, alpha_b, z_l)

L_disk = 0.02944;% Disk side length (m)
R_spool = 0.021;
R_w = L_disk/sqrt(3);

alpha_A = (-R_w*alpha_b*cos(-alpha_r)+z_l)/R_spool;
alpha_B = (-R_w*alpha_b*cos(-alpha_r+2*pi/3)+z_l)/R_spool;
alpha_C = (-R_w*alpha_b*cos(-alpha_r+4*pi/3)+z_l)/R_spool;

== matlab function RLtrot/Act2Angle/Subsystem2/MATLAB Function1 ==
  data: alpha_r input; alpha_A output; alpha_b input; z_l input; alpha_B output; alpha_C output
function [alpha_A, alpha_B, alpha_C]= fcn(alpha_r, alpha_b, z_l)

L_disk = 0.02944;% Disk side length (m)
R_spool = 0.021;
R_w = L_disk/sqrt(3);

alpha_A = (-R_w*alpha_b*cos(-alpha_r)+z_l)/R_spool;
alpha_B = (-R_w*alpha_b*cos(-alpha_r+2*pi/3)+z_l)/R_spool;
alpha_C = (-R_w*alpha_b*cos(-alpha_r+4*pi/3)+z_l)/R_spool;

== matlab function RLtrot/Act2angle/MATLAB Function1 ==
  data: alpha_r input; alpha_A output; alpha_b input; z_l input; alpha_B output; alpha_C output
function [alpha_A, alpha_B, alpha_C]= fcn(alpha_r, alpha_b, z_l)

L_disk = 0.02944;% Disk side length (m)
R_spool = 0.021;
R_w = L_disk/sqrt(3);

alpha_A = (-R_w*alpha_b*cos(-alpha_r)+z_l)/R_spool;
alpha_B = (-R_w*alpha_b*cos(-alpha_r+2*pi/3)+z_l)/R_spool;
alpha_C = (-R_w*alpha_b*cos(-alpha_r+4*pi/3)+z_l)/R_spool;

== matlab function RLtrot/Extropy1/MATLAB Function ==
  data: EntropyWeightList input; EntropyList input; isDone input
function fcn(EntropyWeightList, EntropyList, isDone)
    coder.extrinsic('assignin', 'currentTimestr', 'now', 'evalin', 'datestr');
    if isDone
        xlimEntropy = find(EntropyWeightList,1,'Last')-1;

        figure(5);
        set(gcf,'Visible','on')

        subplot(2,1,1)
        plot(EntropyList(2:end))
        xlabel('Samples')
        ylabel('Expected Entropy')
        xlim([-0.1,xlimEntropy])

        subplot(2,1,2)
        plot(EntropyWeightList(2:end))
        xlabel('Samples')
        ylabel('Entropy Weight')
        xlim([-0.1,xlimEntropy])
        % hold off

        % save the collected data
        evalin('base', 'currentTimestr = datestr(now,''yyyy_mmmm_dd_HH_MM'');');
        evalin('base', 'data.obsv = obsv_vec;');
        evalin('base', 'data.act = act_vec;');
        evalin('base', 'save(append(''Entropy\Entropy_'', currentTimestr,''.mat''), ''data'');');
    end
end

== matlab function RLtrot/Extropy1/MATLAB Function1 ==
  settings: updateMethod=DISCRETE  sampleTime=Ts
  data: time input; obsv input; act input
function store_data(time, obsv, act)
    coder.extrinsic('assignin', 'evalin');
    if time == 0
        assignin("base", "obsv_vec", [ones(1, 10); zeros(100, 10)]);
        assignin("base", "act_vec", [ones(1, 12); zeros(100, 12)]);
        evalin('base', 'clear(''data'');');
    end

    assignin("base", "obsv", obsv');
    assignin("base", "act", act');
    evalin('base', '[rows, ~] = find(obsv_vec, 1, ''last'');');
    evalin('base', 'obsv_vec(rows + 1, :) = obsv;');
    evalin('base', 'act_vec(rows + 1, :) = act;');
